simulink library "Phidgets"  (R2015a)
settings: Solver=ode45  SolverMode=SingleTasking  StartTime=0.0  StopTime=10.0  RelTol=1e-3
settings Model: CovSFcnEnable=off  Creator=test2  LastModifiedBy=uvs
settings DataIOCC: SignalLoggingSaveFormat=ModelDataLogs
settings OptimizationCC: BlockReduction=off  BooleanDataType=off
settings DebuggingCC: SaveWithParameterizedLinksMsg=none  UnderspecifiedInitializationDetection=Classic  MergeDetectMultiDrivingBlocksExec=none  SignalResolutionControl=TryResolveAllWithWarning  MultiTaskCondExecSysMsg=none  StrictBusMsg=None
settings HardwareCC: TargetUnknown=on

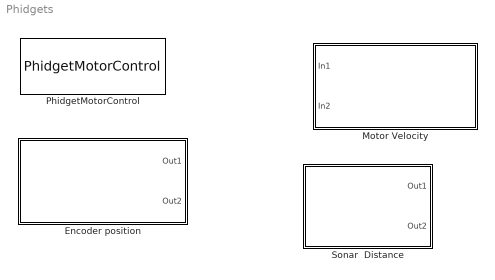
== system Phidgets ==
  Encoder position : Subsystem  mask{Tenc=-1}
      mask prompts: Tenc "Sample time:"
      mask help: This block will retrieve the encoder position of the left and right motors. In order to use this block, a PhidgetMotorControl block must be located in the model and the corresponding serial numbers must be assigned there.
      mask Display:
      | color('red')
      | disp('Encoder Position')
      | port_label('output',1,'Left encoder')
      | port_label('output',2,'Right encoder')
  Motor Velocity : Subsystem  mask{Tmot=-1}
      mask prompts: Tmot "Sample time:"
      mask help: This block will send the velocity command to the left and right motors. In order to use this block, a PhidgetMotorControl block must be located in the model and the corresponding serial numbers must be assigned there.
      mask Display:
      | color('red')
      | disp('Motor Velocity')
      | port_label('input',1,'Left motor')
      | port_label('input',2,'Right motor')
  PhidgetMotorControl : S-Function  FunctionName=PhidgetMotorControl  Parameters=serialLeft,serialRight  mask{serialLeft=-1, serialRight=-1}
      mask prompts: serialLeft "Left:"; serialRight "Right:"
      mask help:
      | This block will initialize left and right PhidgetMotorControl boards with their serial numbers.
      | You can find out the serial numbers of your Phidgets from the Phidget Control Panel on the taskbar after plugging the boards into USB ports.
      | If you leave the Serial Number -1, it will attach to the first Phidget it finds but then using multiple Phidgets may not be possible.
      mask Help: http://www.phidgets.com/docs/Language_-_Simulink#Example_Code
      mask Display:
      | color('red')
      | disp('PhidgetMotorControl')
  Sonar  Distance : Subsystem  mask{Tsensor=0.1}
      mask prompts: Tsensor "Sample Time:"
      mask help: This block will retrieve the distance value measured by the sonar connected to Analog Port 0 of the left and right Phidget boards. In order to use this block, a PhidgetMotorControl block must be located in the model and the corresponding serial numbers must be assigned there.
      mask Display:
      | color('red')
      | disp('Sonar Distance')
      | port_label('output',1,'Left sonar')
      | port_label('output',2,'Right sonar')

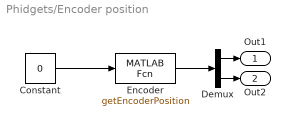
== system Phidgets/Encoder position ==
  Constant : Constant  Value=0
  Demux : Demux  Outputs=2
  Encoder : MATLABFcn  MATLABFcn=getEncoderPosition  OutputDimensions=2  SampleTime=Tenc
  Out1 : Outport
  Out2 : Outport  Port=2
  wires:
  Demux/2 -> Out2/1
  Demux/1 -> Out1/1
  Encoder/1 -> Demux/1
  Constant/1 -> Encoder/1

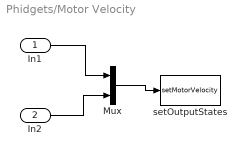
== system Phidgets/Motor Velocity ==
  In1 : Inport
  In2 : Inport  Port=2
  Mux : Mux  Inputs=2
  setOutputStates : MATLABFcn  MATLABFcn=setMotorVelocity  OutputDimensions=0  SampleTime=Tmot
  wires:
  In2/1 -> Mux/2
  Mux/1 -> setOutputStates/1
  In1/1 -> Mux/1

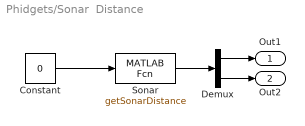
== system Phidgets/Sonar  Distance ==
  Constant : Constant  Value=0
  Demux : Demux  Outputs=2
  Sonar : MATLABFcn  MATLABFcn=getSonarDistance  OutputDimensions=2  SampleTime=Tsensor
  Out1 : Outport
  Out2 : Outport  Port=2
  wires:
  Constant/1 -> Sonar/1
  Demux/2 -> Out2/1
  Demux/1 -> Out1/1
  Sonar/1 -> Demux/1
